simulink model "RefModel_FlightPerf"  (R2020b)
settings: Solver=ode1  StartTime=0.0  StopTime=10.0  FixedStep=SimParam.FightPerf.Ts_base  RelTol=1e-3
(part 2 of 2)

== stateflow chart RefModel_FlightPerf/FlightPerformanceModel/FlightPerf_StateFlow ==
  state FlightPerfPlatform [parallel]
    en:
    initMember();
    initOutputData();
    en,du:
    getTaskData();
    getFlightData();
    getWindData();
    getMavData();
    settings: executionOrder=1
    state LogData [parallel]
      en:
      settings: executionOrder=1
      state Work
        en,du:
        du_func_commonInfo();
        du_func_updateLog();
      (default) -> FlightPerfPlatform.LogData.Work
    state Core [parallel]
      settings: executionOrder=2
      state PowerConsumeByUavMode [parallel]
        settings: executionOrder=1
        state Rotor
          en:
        state Fix
          en:
        (default) -> FlightPerfPlatform.Core.PowerConsumeByUavMode.Rotor
        FlightPerfPlatform.Core.PowerConsumeByUavMode.Rotor -> Fix : [isUavInFix]
        Fix -> FlightPerfPlatform.Core.PowerConsumeByUavMode.Rotor : [isUavInRotor]
      state OverAllParam [parallel]
        settings: executionOrder=2
        state Rotor
          en:
          initFlightPerOut;
          du:
          on every(ceil(0.2/Ts),tick):
          predictDistToFly;
          on every(ceil(1/Ts),tick):
          predictTimeAndPowerToFly(1);
          predictRemainPowerWhenComplete;
          isPowerEnoughToCompleteTask;
        (default) -> FlightPerfPlatform.Core.OverAllParam.Rotor
      state EconomicAirspeed [parallel]
        settings: executionOrder=3
        state Work
          en,du:
          du_func;
        (default) -> FlightPerfPlatform.Core.EconomicAirspeed.Work
  data: flag function_output; period function_input; flag function_output; lla function_input; ll0 function_input; p function_output; blockName function_input; message function_input; operation function_input; varargin function_input; success function_output; message_in function_input; varargin function_input; debugInfo function_input; tabspace function_input; varargin function_input; modeName function_input; debugInfo function_input; varargin function_input; clock_sec input; isDebugInfoToShow input; Ts input; IN_TaskCmd input Bus: BUS_TASK_PATH_OutParam size=1; IN_FlightParam input Bus: BUS_TASK_COMMON_OutParam size=1; mission_item_def input Bus: mavlink_mission_item_def size=TASK_PARAM_V1000.maxPathPointNum; TaskParam data_store_memory; FlightPerfParam data_store_memory size=1; FlightPerfOut output Bus: BUS_FLIGHTPERF_OUT size=1; mavlink_msg_command_battery_data input Bus: mavlink_msg_command_battery_data size=1; mavlink_msg_mission_current input Bus: mavlink_msg_mission_current; IN_WindNED input; TimeSpend local; logDataBuffer output Bus: BUS_FLIGHTPERF_SingleLog size=32; logDataOut output Bus: BUS_FLIGHTPERF_SingleLog size=1; mTask_taskMode local; mTask_currentPointNum local =2; mTask_validPathNum local; mTask_uavMode local; mTask_heightSwitchMode local; mFParam_LLA local; mFParam_WindSpeed local; mFParam_HomeLLA local; mFParam_altitude local; mWind_WindSpeed local; mWind_WindHeading local; mMav_batteryLife local =0
  function initOutputData:
    | function initOutputData
    | % 输出结构体进行赋值，避免报"调用前没有赋值"的错误，每个结构体赋值1个成员即可
    | logDataOut(1).time_sec = 0;
    | logDataBuffer(1).time_sec = 0;
  function initMember:
    | function initMember()
    | % 初始化成员变量
    | mTask_currentPointNum = 0;
    | mTask_validPathNum = 0;
  function getTaskData:
    | function getTaskData()
    | %% 输入结构体
    | %% 直接量
    | mTask_taskMode = IN_TaskCmd.flightTaskMode;
    | mTask_currentPointNum = IN_TaskCmd.currentPointNum;
    | mTask_validPathNum = IN_TaskCmd.validPathNum;
    | mTask_uavMode = IN_TaskCmd.uavMode;
    | mTask_heightSwitchMode = IN_TaskCmd.heightSwitchMode;
    | %% 间接量
  function getMavData:
    | function getMavData()
    | %% 输入结构体
    | %% 直接量
    | mMav_batteryLife = getLowestBatteryLife(); %double(mavlink_msg_mission_current(1).remaining);
    | %% 间接量
    | 
    | %% 子函数 ------------------------------------------------------------
    | function minLife = getLowestBatteryLife()
    | persistent du
    | if isempty(du)
    |     du = 0;
    | end
    | out = 0;
    | du = du + Ts;
    | nIter = TaskParam.maxNumBattery;
    | nValid = TaskParam.nBattery;
    | flagAllZero = true;
    | minLife = 100;
    | for i = 1:nIter
    |     if i <= nValid
    |         thisLife = double(mavlink_msg_mission_current(i).remaining);
    |         if thisLife > 1e-6 % 非零
    |             flagAllZero = false;
    |             minLife = min(minLife,thisLife);
    |         end
    |     end
    | end
    | % if flagAllZero && du > 1
    | %     du = 0;
    | %     runLog(ENUM_RTInfo_Task.BatteryInfo_AllZero,[0,0,0,0,0]);
    | % end
  function getFlightData:
    | function getFlightData()
    | %% 输入结构体
    | %% 直接量
    | mFParam_LLA = IN_FlightParam.curLLA;
    | mFParam_WindSpeed = IN_FlightParam.curWindSpeedFromHead;
    | mFParam_HomeLLA = IN_FlightParam.curHomeLLA;
    | mFParam_altitude = IN_FlightParam.altitude;
    | %% 间接量
  function getWindData:
    | function getWindData()
    | %% 输入结构体
    | %% 直接量
    | mWind_WindSpeed = IN_WindNED.windSpeed_ms;
    | mWind_WindHeading = IN_WindNED.windHeading_rad;
    | %% 间接量
  function du_func_commonInfo:
    | function du_func_commonInfo
  function du_func_updateLog:
    | function du_func_updateLog
    | updateLogDataBuffer(ENUM_FlightPerfLogBlockName.FPLOG_None,ENUM_RTInfo_FlightPerf(0),'read')
  function predictRemainPowerWhenComplete:
    | function predictRemainPowerWhenComplete()
    | FlightPerfOut.remainPowerWhenFinish_per = mMav_batteryLife - FlightPerfOut.batteryLifeToCompleteTask;
  function predictDistToFly:
    | function predictDistToFly
    | persistent hasTakeOff remainDistToGo_movsmooth hasBeginGoHome
    | if isempty(hasTakeOff)
    |     hasTakeOff = false;
    |     hasBeginGoHome = false;
    |     remainDistToGo_movsmooth = 0;
    | end
    | if mTask_validPathNum == 0
    |     FlightPerfOut.remainDistToGo_m = 0;
    |     return;
    | end
    | validNum = 0;
    | maxNum = length(mission_item_def);
    | % 
    | nanFlag = TaskParam.nanFlag;
    | if isDataRefresh(mission_item_def,maxNum,nanFlag) % 检测航点是否更新
    |     refreshFlag = true;
    | else
    |     refreshFlag = false;
    | end
    | % 当前目标航点
    | if mTask_currentPointNum ~= 0 % 进入航线模式前
    |     idxCur = mTask_currentPointNum;
    | else
    |     idxCur = 2;
    | end
    | curPathPoint = double([mission_item_def(idxCur).x,mission_item_def(idxCur).y, mission_item_def(idxCur).z]);
    | % 最后一个航点
    | if mTask_validPathNum ~= 0
    |     idxLast = mTask_validPathNum;
    | else
    |     idxLast = 3;
    | end
    | lastValidPathPoint = double([mission_item_def(idxLast).x,mission_item_def(idxLast).y, mission_item_def(idxLast).z]);
    | % home点
    | idxHome = 1;
    | homePoint = double([mission_item_def(idxHome).x,mission_item_def(idxHome).y, mission_item_def(idxHome).z]);
    | % 当前位置
    | curLLA = mFParam_LLA;
    | %
    | % FlightPerfOut.remainDistToGo_m = 0;
    | if mTask_taskMode == ENUM_FlightTaskMode.TakeOffMode
    |     hasTakeOff = true;
    | end
    | if mTask_taskMode == ENUM_FlightTaskMode.GoHomeMode
    |     hasBeginGoHome = true;
    | end
    | %
    | switch mTask_taskMode
    |     case ENUM_FlightTaskMode.GroundStandByMode
    |         if hasTakeOff
    |             FlightPerfOut.remainDistToGo_m = 0;
    |         else
    |             idxStart = 1;
    |             restAllPath = calDistFromCurToHome(idxCur,maxNum,mTask_validPathNum,mission_item_def,FlightPerfParam,refreshFlag);
    |             tempPos = lla2ned(curLLA, curPathPoint(1:2));
    |             distToCurPathPoint = norm(tempPos(1:2));
    |             tempPos = lla2ned(lastValidPathPoint, homePoint(1:2));
    |             distFromEndPointToHome = norm(tempPos(1:2));
    |             FlightPerfOut.remainDistToGo_m = restAllPath + distToCurPathPoint + distFromEndPointToHome + 200;
    |         end
    |     case {  ENUM_FlightTaskMode.TakeOffMode,...
    |             ENUM_FlightTaskMode.HoverUpMode,...
    |             ENUM_FlightTaskMode.Rotor2Fix_Mode}
    |         modeflag = 'beforePathMode';
    |         idxStart = 1;
    |         restAllPath = calDistFromCurToHome(idxCur,maxNum,mTask_validPathNum,mission_item_def,FlightPerfParam,refreshFlag);
    |         tempPos = lla2ned(curLLA, curPathPoint(1:2));
    |         distToCurPathPoint = norm(tempPos(1:2));
    |         tempPos = lla2ned(lastValidPathPoint, homePoint(1:2));
    |         distFromEndPointToHome = norm(tempPos(1:2));
    |         FlightPerfOut.remainDistToGo_m = restAllPath + distToCurPathPoint + distFromEndPointToHome + 200;
    |     case {ENUM_FlightTaskMode.PathFollowMode,...
    |             ENUM_FlightTaskMode.AirStandByMode}
    |         modeflag = 'duringPathMode';
    |         idxStart = 2;
    |         restAllPath = calDistFromCurToHome(idxCur,maxNum,mTask_validPathNum,mission_item_def,FlightPerfParam,refreshFlag);
    |         tempPos = lla2ned(curLLA, curPathPoint(1:2));
    |         distToCurPathPoint = norm(tempPos(1:2));
    |         tempPos = lla2ned(lastValidPathPoint, homePoint(1:2));
    |         distFromEndPointToHome = norm(tempPos(1:2));
    |         FlightPerfOut.remainDistToGo_m = restAllPath + distToCurPathPoint + distFromEndPointToHome;
    |         if hasBeginGoHome && ...
    |                 mTask_taskMode == ENUM_FlightTaskMode.AirStandByMode
    |             FlightPerfOut.remainDistToGo_m = distToCurPathPoint;
    |         end
    |     case ENUM_FlightTaskMode.GoHomeMode
    |         modeflag = 'GoHomeMode';
    |         tempPos = lla2ned(curLLA, homePoint(1:2));
    |         distFromCurLLAToHome = norm(tempPos(1:2));
    |         FlightPerfOut.remainDistToGo_m = distFromCurLLAToHome;
    |     otherwise
    |         modeflag = 'afterHomeMode';
    | end
    | FlightPerfOut.remainDistToGo_m = movsmooth(FlightPerfOut.remainDistToGo_m);
    | end
    | %% 子函数
    | function flag = isDataRefresh(pathdata,maxNum,nanFlag)
    | persistent preSum
    | if isempty(preSum)
    |     preSum = 0;
    | end
    | flag = false;
    | sum = 0;
    | for i = 2:maxNum % 从第2个数据点开始，不考虑home点
    |     if pathdata(i).x ~= nanFlag
    |         sum = sum + double(i*pathdata(i).x + 1.1*i*pathdata(i).y);
    |     end
    | end
    | if preSum ~= sum
    |     flag = true;
    | end
    | preSum = sum;
    | end
    | 
    | function [remainDistToGo_m] = calDistFromCurToHome(curNum,maxNum,validNum,mission_item_def,FlightPerfParam,refreshFlag)
    | % 从当前位置算起，完成剩余航点后返回到home点的总距离
    |     persistent isPathValid isCalComplete pathDistSet
    |     if isempty(isPathValid)
    |         isPathValid = false;
    |         isCalComplete = false;
    |         pathDistSet = zeros(1,maxNum);
    |     end
    |     if validNum >= 2 && (~isCalComplete || refreshFlag) 
    |         isPathValid = true;
    |         for idx = curNum:maxNum-1
    |             tempPrePathPoint = double([mission_item_def(idx).x,mission_item_def(idx).y, mission_item_def(idx).z]);
    |             tempCurPathPoint = double([mission_item_def(idx+1).x,mission_item_def(idx+1).y, mission_item_def(idx+1).z]);
    |             tempPos = lla2ned(tempPrePathPoint, tempCurPathPoint(1:2));
    |             tempDist = norm(tempPos(1:2));
    |             if idx <= validNum-1
    |                 pathDistSet(idx) = tempDist;
    |             else
    |                 break;
    |             end
    |         end
    |         isCalComplete = true;
    |     end
    |     modeSel = 'pre_cal'; % rt_cal pre_cal  实时计算or预计算
    |     switch modeSel
    |         case 'rt_cal'
    |             if curNum ~= 0 % 进入航线模式前
    |                 idxCur = curNum;
    |             else
    |                 idxCur = 2;
    |             end
    |             curPathPoint = double([mission_item_def(idxCur).x,mission_item_def(idxCur).y, mission_item_def(idxCur).z]);
    |             remainDistToGo_m = 0;
    |             remainPathPoint = 0;
    |             for idx = curNum:maxNum-1
    |                 tempPrePathPoint = double([mission_item_def(idx).x,mission_item_def(idx).y, mission_item_def(idx).z]);
    |                 tempCurPathPoint = double([mission_item_def(idx+1).x,mission_item_def(idx+1).y, mission_item_def(idx+1).z]);
    |                 tempPos = lla2ned(tempPrePathPoint, tempCurPathPoint(1:2));
    |                 tempDist = norm(tempPos(1:2));
    |                 if idx <= validNum-1 && isPathPointValid(curPathPoint)
    |                     remainDistToGo_m = remainDistToGo_m + tempDist + FlightPerfParam.addedDistByEachTurnCorrect;
    |                 else
    |                     break;
    |                 end
    |             end
    |         otherwise
    |             nPoint = validNum - curNum;
    |             remainDistToGo_m = sum(pathDistSet(curNum:end)) + nPoint*FlightPerfParam.addedDistByEachTurnCorrect;
    |     end
    | end
    | %
    | function out = movsmooth(val)
    | persistent valsmooth
    | if isempty(valsmooth)
    |     valsmooth = 0;
    | end
    | if val ~= 0
    |     %     if norm(valsmooth-val)<2000
    |     kscale = 11/12;
    |     valsmooth = kscale*valsmooth + (1-kscale)*val;
    |     out = valsmooth;
    |     %     else
    |     %         out = val;
    |     %     end
    | else
    |     out = 0;
    | end
    | end
    | %
    | function flag = isPathPointValid(LLA)
    | flag = true;
    | for i_LLA = 1:2
    |     if abs(LLA(i_LLA)) > 360
    |         flag = false;
    |     end
    | end
    | end
  function flag = isUavInRotor:
    | function flag = isUavInRotor
    | flag = false;
    | if mTask_uavMode == ENUM_UAVMode.Rotor
    |     flag = true;
    | end
  function isPowerEnoughToCompleteTask:
    | function isPowerEnoughToCompleteTask
    | if FlightPerfOut.remainPowerWhenFinish_per <= FlightPerfParam.reservedPowerRate_normal %TaskParam.low_battery_alarm_set
    |     FlightPerfOut.isAbleToCompleteTask = false;
    | else 
    |     FlightPerfOut.isAbleToCompleteTask = true;
    | end
  function predictTimeAndPowerToFly(period):
    | function predictTimeAndPowerToFly(period)
    | persistent preTimeSpend preBatterySpend hasEnterLandMode hasEnterHoverDown hasBeenInPath hasVerticalMoveBeforePath hasVerticalMoveBeforeHome
    | if isempty(preTimeSpend)
    |     preTimeSpend = 0;
    |     preBatterySpend = 0;
    |     hasEnterHoverDown = false;
    |     hasEnterLandMode = false;
    |     hasBeenInPath = false;
    |     hasVerticalMoveBeforePath = false;
    |     hasVerticalMoveBeforeHome = false;
    | end
    | if FlightPerfOut.remainDistToGo_m == 0
    |     FlightPerfOut.remainTimeToSpend_sec = 0;
    |     return;
    | end
    | % 海拔、风等因素对续航的修正系数
    | k_Alt = calHeightScaleForPowerConsum();
    | kTakeOff_AltCorrect = 1.15*k_Alt;
    | kPath_AltCorrect = 1.15*k_Alt;
    | kLand_AltCorrect = 1.15*k_Alt;
    | kLand_WindCorrect = 1+abs(mWind_WindSpeed)/15; % 当风速15m/s时, 系数为 2
    | %
    | timeSpend = 0; % 完成任务所需时间
    | 
    | switchHeight = mTask_heightSwitchMode; % 固定翼切换高度
    | curHeight = mFParam_LLA(3);
    | homeHeight = double(mission_item_def(1).z); % home高度，注意，等高航线中home点高度存在高于航线高度的情况
    | pathHeight = double(mission_item_def(2).z); % 航线高度 ！V1000仅有等高航线，若后续增加变高航线，该处可能需调整
    | errHeight_Home_Path = abs(homeHeight-pathHeight);
    | errHeight_Cur_Path = abs(curHeight-pathHeight);
    | errHeight_Cur_Home = abs(curHeight-homeHeight);
    | % 模式耗时
    | timeSpend_TakeOff = 15 + switchHeight/(TaskParam.maxClimbSpeed_normal_TakeOffandLand+eps);
    | timeSpend_HoverAfterTakeOff = 10;
    | timeSpend_Rotor2Fix = 10;
    | timeSpend_HoverUp = abs(homeHeight-switchHeight)/(TaskParam.maxClimbSpeed_fixMode+eps);
    | timeSpend_VerticalMoveBeforePath = errHeight_Home_Path/(TaskParam.maxClimbSpeed_fixMode+eps);
    | timeSpend_Path = FlightPerfOut.remainDistToGo_m/(TaskParam.cruiseSpeed_cruise+eps)+FlightPerfOut.remainPathPoint*15;
    | timeSpend_VerticalMoveBeforeGoHome = errHeight_Home_Path/(TaskParam.maxClimbSpeed_fixMode+eps);
    | timeSpend_HoverDown = timeSpend_HoverUp + 25;
    | timeSpend_Fix2Rotor = 10;
    | timeSpend_GoHome_Rotor_full = 100/TaskParam.cruiseSpeed_rotorMode;
    | timeSpend_GoHome_Rotor_part = FlightPerfOut.remainDistToGo_m/TaskParam.cruiseSpeed_rotorMode;
    | timeSpend_Land = kLand_WindCorrect*kLand_AltCorrect*timeSpend_TakeOff;
    | timeSpend_LandFromHomeHeight_ByRotor = kLand_WindCorrect*kLand_AltCorrect*curHeight/(TaskParam.maxClimbSpeed_normal_TakeOffandLand+eps);
    | 
    | batteryLifeSpend_TakeOff = kTakeOff_AltCorrect*timeSpend_TakeOff*FlightPerfParam.powerRate_RotorUpNoWind;
    | batteryLifeSpend_HoverAfterTakeOff = timeSpend_HoverAfterTakeOff*FlightPerfParam.powerRate_RotorHoverNoWind;
    | batteryLifeSpend_Rotor2Fix = timeSpend_Rotor2Fix*FlightPerfParam.powerRate_RotorHoverNoWind;
    | batteryLifeSpend_HoverUp = timeSpend_HoverUp*FlightPerfParam.powerRate_FixHoverUp;
    | batteryLifeSpend_VerticalMoveBeforePath = timeSpend_VerticalMoveBeforePath*FlightPerfParam.powerRate_FixHoverDown;
    | batteryLifeSpend_Path = kPath_AltCorrect*timeSpend_Path*FlightPerfParam.powerRate_FixCruise;
    | batteryLifeSpend_VerticalMoveBeforeGoHome = timeSpend_VerticalMoveBeforeGoHome*FlightPerfParam.powerRate_FixHoverUp;
    | batteryLifeSpend_HoverDown = timeSpend_HoverDown*FlightPerfParam.powerRate_FixHoverDown;
    | batteryLifeSpend_Fix2Rotor = timeSpend_Fix2Rotor*FlightPerfParam.powerRate_RotorUpNoWind;
    | batteryLifeSpend_GoHome_Rotor_full = timeSpend_GoHome_Rotor_full*FlightPerfParam.powerRate_RotorMoveNoWind;
    | batteryLifeSpend_GoHome_Rotor_part = timeSpend_GoHome_Rotor_part*FlightPerfParam.powerRate_RotorMoveNoWind;
    | batteryLifeSpend_Land = timeSpend_Land*FlightPerfParam.powerRate_RotorDownNoWind;
    | batteryLifeSpend_LandFromHomeHeight_ByRotor = timeSpend_LandFromHomeHeight_ByRotor*FlightPerfParam.powerRate_RotorDownNoWind;
    | 
    | if mTask_taskMode == ENUM_FlightTaskMode.LandMode
    |     hasEnterLandMode = true;
    | end
    | if mTask_taskMode == ENUM_FlightTaskMode.HoverDownMode
    |     hasEnterHoverDown = true;
    | end
    | if mTask_taskMode == ENUM_FlightTaskMode.VerticalMove
    |     hasVerticalMoveBeforePath = true;
    | end
    | if mTask_currentPointNum > 2
    |     hasBeenInPath = true;
    | end
    | if mTask_taskMode == ENUM_FlightTaskMode.VerticalMove && hasBeenInPath
    |     hasVerticalMoveBeforeHome = true;
    | end
    | switch mTask_taskMode
    |     case ENUM_FlightTaskMode.GroundStandByMode
    |         if hasEnterLandMode
    |             timeSpend = 0;
    |             batterySpend = 0;
    |         else
    |             timeSpend = ...
    |                 timeSpend_TakeOff + ...
    |                 timeSpend_HoverAfterTakeOff + ...
    |                 timeSpend_Rotor2Fix + ...
    |                 timeSpend_HoverUp + ...
    |                 timeSpend_VerticalMoveBeforePath + ...
    |                 timeSpend_Path + ...
    |                 timeSpend_VerticalMoveBeforeGoHome + ...
    |                 timeSpend_HoverDown + ...
    |                 timeSpend_Fix2Rotor + ...
    |                 timeSpend_GoHome_Rotor_full + ...
    |                 timeSpend_Land;
    |             batterySpend = ...
    |                 batteryLifeSpend_TakeOff + ...
    |                 batteryLifeSpend_HoverAfterTakeOff + ...
    |                 batteryLifeSpend_Rotor2Fix + ...
    |                 batteryLifeSpend_HoverUp + ...
    |                 batteryLifeSpend_VerticalMoveBeforePath + ...
    |                 batteryLifeSpend_Path + ...
    |                 batteryLifeSpend_VerticalMoveBeforeGoHome + ...
    |                 batteryLifeSpend_HoverDown + ...
    |                 batteryLifeSpend_Fix2Rotor + ...
    |                 batteryLifeSpend_GoHome_Rotor_full + ...
    |                 batteryLifeSpend_Land;
    |         end
    |     case ENUM_FlightTaskMode.TakeOffMode
    |         timeSpend = ...
    |             timeSpend_Rotor2Fix + ...
    |             timeSpend_HoverUp + ...
    |             timeSpend_VerticalMoveBeforePath + ...
    |             timeSpend_Path + ...
    |             timeSpend_VerticalMoveBeforeGoHome + ...
    |             timeSpend_HoverDown + ...
    |             timeSpend_Fix2Rotor + ...
    |             timeSpend_GoHome_Rotor_full + ...
    |             timeSpend_Land;
    |         batterySpend = ...
    |             batteryLifeSpend_Rotor2Fix + ...
    |             batteryLifeSpend_HoverUp + ...
    |             batteryLifeSpend_VerticalMoveBeforePath + ...
    |             batteryLifeSpend_Path + ...
    |             batteryLifeSpend_VerticalMoveBeforeGoHome + ...
    |             batteryLifeSpend_HoverDown + ...
    |             batteryLifeSpend_Fix2Rotor + ...
    |             batteryLifeSpend_GoHome_Rotor_full + ...
    |             batteryLifeSpend_Land;
    |         timeByThisTask = 10 + max(0,switchHeight-curHeight)/(TaskParam.maxClimbSpeed_normal_TakeOffandLand+eps);
    |         timeSpend = timeSpend + timeByThisTask;
    |         batterySpendByThisTask = kTakeOff_AltCorrect*timeByThisTask*FlightPerfParam.powerRate_RotorUpNoWind;
    |         batterySpend = batterySpend + batterySpendByThisTask;
    |     case ENUM_FlightTaskMode.HoverUpMode
    |         timeSpend = ...
    |             timeSpend_VerticalMoveBeforePath + ...
    |             timeSpend_Path + ...
    |             timeSpend_VerticalMoveBeforeGoHome + ...
    |             timeSpend_HoverDown + ...
    |             timeSpend_Fix2Rotor + ...
    |             timeSpend_GoHome_Rotor_full + ...
    |             timeSpend_Land;
    |         batterySpend = ...
    |             batteryLifeSpend_VerticalMoveBeforePath + ...
    |             batteryLifeSpend_Path + ...
    |             batteryLifeSpend_VerticalMoveBeforeGoHome + ...
    |             batteryLifeSpend_HoverDown + ...
    |             batteryLifeSpend_Fix2Rotor + ...
    |             batteryLifeSpend_GoHome_Rotor_full + ...
    |             batteryLifeSpend_Land;
    |         timeByThisTask = 10 + max(0,homeHeight-curHeight)/(TaskParam.maxClimbSpeed_fixMode+eps);
    |         timeSpend = timeSpend + timeByThisTask;
    |         batterySpendByThisTask = timeByThisTask*FlightPerfParam.powerRate_FixHoverUp;
    |         batterySpend = batterySpend + batterySpendByThisTask;
    |     case ENUM_FlightTaskMode.VerticalMove
    |         if hasVerticalMoveBeforePath && ~hasVerticalMoveBeforeHome
    |             % 从home高度降至path高度
    |             timeSpend = ...
    |                 timeSpend_Path + ...
    |                 timeSpend_VerticalMoveBeforeGoHome + ...
    |                 timeSpend_HoverDown + ...
    |                 timeSpend_Fix2Rotor + ...
    |                 timeSpend_GoHome_Rotor_full + ...
    |                 timeSpend_Land;
    |             timeSpend_VerticalMoveBeforePath_RT = errHeight_Cur_Path/(TaskParam.maxClimbSpeed_fixMode+eps);
    |             timeSpend = timeSpend + timeSpend_VerticalMoveBeforePath_RT;
    |             batterySpend = ...
    |                 batteryLifeSpend_Path + ...
    |                 batteryLifeSpend_VerticalMoveBeforeGoHome + ...
    |                 batteryLifeSpend_HoverDown + ...
    |                 batteryLifeSpend_Fix2Rotor + ...
    |                 batteryLifeSpend_GoHome_Rotor_full + ...
    |                 batteryLifeSpend_Land;
    |             batterySpend = batterySpend + timeSpend_VerticalMoveBeforePath_RT*FlightPerfParam.powerRate_FixHoverDown;
    |         else % if hasVerticalMoveBeforePath
    |             % 从path高度上升至home高度
    |             timeSpend = ...
    |                 timeSpend_Path + ...
    |                 timeSpend_HoverDown + ...
    |                 timeSpend_Fix2Rotor + ...
    |                 timeSpend_GoHome_Rotor_full + ...
    |                 timeSpend_Land;
    |             timeSpend_VerticalMoveBeforeGoHome_RT = errHeight_Cur_Home/(TaskParam.maxClimbSpeed_fixMode+eps);
    |             timeSpend = timeSpend + timeSpend_VerticalMoveBeforeGoHome_RT;
    |             batterySpend = ...
    |                 batteryLifeSpend_Path + ...
    |                 batteryLifeSpend_HoverDown + ...
    |                 batteryLifeSpend_Fix2Rotor + ...
    |                 batteryLifeSpend_GoHome_Rotor_full + ...
    |                 batteryLifeSpend_Land;
    |             batterySpend = batterySpend + timeSpend_VerticalMoveBeforeGoHome_RT*FlightPerfParam.powerRate_FixHoverUp;
    |         end
    |     case ENUM_FlightTaskMode.PathFollowMode
    |         timeSpend = ...
    |             timeSpend_Path + ...
    |             timeSpend_HoverDown + ...
    |             timeSpend_Fix2Rotor + ...
    |             timeSpend_GoHome_Rotor_full + ...
    |             timeSpend_Land;
    |         batterySpend = ...
    |             batteryLifeSpend_Path + ...
    |             batteryLifeSpend_HoverDown + ...
    |             batteryLifeSpend_Fix2Rotor + ...
    |             batteryLifeSpend_GoHome_Rotor_full + ...
    |             batteryLifeSpend_Land;
    |         if ~hasVerticalMoveBeforePath
    |             timeSpend = timeSpend + timeSpend_VerticalMoveBeforePath + timeSpend_VerticalMoveBeforeGoHome;
    |             batterySpend = batterySpend + ...
    |                 batteryLifeSpend_VerticalMoveBeforePath + ...
    |                 batteryLifeSpend_VerticalMoveBeforeGoHome;
    |         elseif hasVerticalMoveBeforePath && ~hasVerticalMoveBeforeHome
    |             timeSpend_VerticalMoveBeforePath_RT = errHeight_Cur_Path/(TaskParam.maxClimbSpeed_fixMode+eps);
    |             timeSpend = timeSpend + timeSpend_VerticalMoveBeforePath_RT + timeSpend_VerticalMoveBeforeGoHome;
    |             batterySpend = batterySpend + ...
    |                 timeSpend_VerticalMoveBeforePath_RT*FlightPerfParam.powerRate_FixHoverDown + ...
    |                 batteryLifeSpend_VerticalMoveBeforeGoHome;
    |         elseif hasVerticalMoveBeforeHome
    |             timeSpend_VerticalMoveBeforeGoHome_RT = errHeight_Cur_Home/(TaskParam.maxClimbSpeed_fixMode+eps);
    |             timeSpend = timeSpend + timeSpend_VerticalMoveBeforeGoHome_RT;
    |             batterySpend = batterySpend + ...
    |                 timeSpend_VerticalMoveBeforeGoHome_RT*FlightPerfParam.powerRate_FixHoverDown;
    |         end
    |     case ENUM_FlightTaskMode.GoHomeMode
    |         if ~hasEnterHoverDown
    |             timeSpend = ...
    |                 timeSpend_Path + ...
    |                 timeSpend_HoverDown + ...
    |                 timeSpend_Fix2Rotor + ...
    |                 timeSpend_GoHome_Rotor_full + ...
    |                 timeSpend_Land;
    |             batterySpend = ...
    |                 batteryLifeSpend_Path + ...
    |                 batteryLifeSpend_HoverDown + ...
    |                 batteryLifeSpend_Fix2Rotor + ...
    |                 batteryLifeSpend_GoHome_Rotor_full + ...
    |                 batteryLifeSpend_Land;
    |         else
    |             timeSpend = ...
    |                 timeSpend_GoHome_Rotor_part + ...
    |                 timeSpend_Land;
    |             batterySpend = ...
    |                 batteryLifeSpend_GoHome_Rotor_part + ...
    |                 batteryLifeSpend_Land;
    |         end
    |     case ENUM_FlightTaskMode.HoverDownMode
    |         if abs(curHeight-switchHeight) > 10
    |             % 盘旋下降（不考虑滑翔方式的节能影响，让按照正常耗电计算）
    |             timeSpend = ...
    |                 timeSpend_Fix2Rotor + ...
    |                 timeSpend_GoHome_Rotor_full + ...
    |                 timeSpend_Land;
    |             batterySpend = ...
    |                 batteryLifeSpend_Fix2Rotor + ...
    |                 batteryLifeSpend_GoHome_Rotor_full + ...
    |                 batteryLifeSpend_Land;
    |             timeByThisTask = abs(curHeight-switchHeight)/(TaskParam.maxClimbSpeed_fixMode+eps)+20;
    |             timeSpend = timeSpend + timeByThisTask;
    |             batterySpendByThisTask = timeByThisTask*FlightPerfParam.powerRate_FixHoverDown;
    |             batterySpend = batterySpend + batterySpendByThisTask;
    |         else
    |             % 盘旋一圈
    |             timeSpend = preTimeSpend - period;
    |             batterySpend = preBatterySpend - period*FlightPerfParam.powerRate_FixHoverLevel;
    |         end
    |     case ENUM_FlightTaskMode.LandMode
    |         if curHeight-10 > 0
    |             timeSpend = (curHeight-10)/(TaskParam.maxClimbSpeed_normal_TakeOffandLand+eps) + 10/TaskParam.maxClimbSpeed_nearGround_TakeOffandLand;
    |         else
    |             timeSpend = curHeight/TaskParam.maxClimbSpeed_nearGround_TakeOffandLand;
    |         end
    |         batterySpend = timeSpend*FlightPerfParam.powerRate_RotorDownNoWind;
    |     case ENUM_FlightTaskMode.Fix2Rotor_Mode
    |         timeSpend = preTimeSpend - period;
    |         batterySpend = preBatterySpend - period*FlightPerfParam.powerRate_RotorHoverNoWind;
    |     case ENUM_FlightTaskMode.Rotor2Fix_Mode
    |         timeSpend = preTimeSpend - period;
    |         batterySpend = preBatterySpend - period*FlightPerfParam.powerRate_RotorHoverNoWind;
    |     case {ENUM_FlightTaskMode.HoverAdjustMode,...
    |             ENUM_FlightTaskMode.AirStandByMode}
    |         timeSpend = preTimeSpend;
    |         batterySpend = preBatterySpend;
    |     otherwise
    |         timeSpend = preTimeSpend;
    |         batterySpend = preBatterySpend;
    | end
    | %% 电量低返航触发标志
    | % 计算风因素对飞行地速的影响
    | homeLLA = mFParam_HomeLLA;
    | curLLA = mFParam_LLA;
    | homeNED = lla2ned(homeLLA,curLLA);
    | curLLA = [0 0 0];
    | headingGoHome_rad = atan2(homeNED(2),homeNED(1));
    | headingErr = angdiff(mWind_WindHeading,headingGoHome_rad);
    | windSpeedWhenGoHomeAtThisLL = mWind_WindSpeed*cos(headingErr); % 正值表示逆风, 负值表示顺风
    | windSpeedWhenGoHomeAtThisLL = min(windSpeedWhenGoHomeAtThisLL,14); % 限制小于14
    | windSpeedWhenGoHomeAtThisLL = max(windSpeedWhenGoHomeAtThisLL,-5); % 限制大于-5
    | 
    | velScale_FixGoHome = 1;
    | speedmode = 'fixAirspeed';
    | switch speedmode
    |     case 'fixAirspeed'
    |         velScale_FixGoHome = TaskParam.cruiseSpeed_cruise / abs(TaskParam.cruiseSpeed_cruise-windSpeedWhenGoHomeAtThisLL);
    | %         velScale_FixGoHome1 = TaskParam.cruiseSpeed_cruise / abs(TaskParam.cruiseSpeed_cruise-windSpeedWhenGoHomeAtThisLL1);
    | %         fprintf('(%.2f) velScale_FixGoHome: %.2f\t\tvelScale_FixGoHome1: %.2f\n',clock_sec,velScale_FixGoHome,velScale_FixGoHome1);
    |     case 'variableAirspeed'
    |         velScale_FixGoHome = 1 + windSpeedWhenGoHomeAtThisLL/TaskParam.cruiseSpeed_cruise;
    | end
    | velScale_RotorGoHome = velScale_FixGoHome;
    | % 注意"盘旋下降、降落、固定翼转旋翼"不进行判断，因为盘旋下降已经处于降落流程且盘旋下降模式耗电量极低
    | % if mTask_taskMode == ENUM_FlightTaskMode.PathFollowMode || ...
    | %         mTask_taskMode == ENUM_FlightTaskMode.GoHomeMode || ...
    | %         mTask_taskMode == ENUM_FlightTaskMode.AirStandByMode || ...
    | %         mTask_taskMode == ENUM_FlightTaskMode.HoverAdjustMode
    | if mTask_taskMode ~= ENUM_FlightTaskMode.GroundStandByMode && ...
    |         mTask_taskMode ~= ENUM_FlightTaskMode.HoverDownMode && ...
    |         mTask_taskMode ~= ENUM_FlightTaskMode.Rotor2Fix_Mode && ...
    |         mTask_taskMode ~= ENUM_FlightTaskMode.LandMode && ...
    |         mTask_taskMode ~= ENUM_FlightTaskMode.NoneFlightTaskMode
    |     % 计算当前点到Home点距离
    |     curLLA = mFParam_LLA;
    |     idxHome = 1;
    |     homeLLA = double([mission_item_def(idxHome).x,mission_item_def(idxHome).y, mission_item_def(idxHome).z]);
    |     tempPos = lla2ned(curLLA, homeLLA(1:2));
    |     distFromCurToHome = norm(tempPos(1:2));
    |     [FlightPerfOut.batterylifeNeededToHome,FlightPerfOut.batterylifeNeededToLand] = batteryLifeToHome(distFromCurToHome,mTask_uavMode,...
    |         batteryLifeSpend_HoverDown,batteryLifeSpend_Fix2Rotor,batteryLifeSpend_GoHome_Rotor_full,batteryLifeSpend_Land,batteryLifeSpend_LandFromHomeHeight_ByRotor,velScale_FixGoHome,velScale_RotorGoHome);
    |     extraLifeNeededByWind = 1/3*abs(mWind_WindSpeed);
    |     if (FlightPerfOut.batterylifeNeededToHome + extraLifeNeededByWind) >= mMav_batteryLife - FlightPerfParam.reservedPowerRate_normal
    |         FlightPerfOut.flagGoHomeNow = true;
    | %         if isDebugInfoToShow
    | %             fprintf('%.3f sec: [flagGoHomeNow] TaskMode(%d) ',clock_sec,mTask_taskMode,) 
    | %         end
    |     end
    |     if (FlightPerfOut.batterylifeNeededToLand + extraLifeNeededByWind) >= mMav_batteryLife - FlightPerfParam.reservedPowerRate_rotor && ...
    |             mTask_uavMode == ENUM_UAVMode.Rotor % (mTask_uavMode == ENUM_UAVMode.Rotor || mTask_uavMode == ENUM_UAVMode.Fix)
    |         % 目前仅在旋翼模式下判断该值，存在逻辑缺陷
    |         FlightPerfOut.flagLandNow = true;
    |     end
    | end
    | %%
    | FlightPerfOut.remainTimeToSpend_sec = double(timeSpend);
    | FlightPerfOut.batteryLifeToCompleteTask = double(batterySpend);
    | preTimeSpend = double(FlightPerfOut.remainTimeToSpend_sec);
    | preBatterySpend = FlightPerfOut.batteryLifeToCompleteTask;
    | end
    | %% 子函数
    | % 计算耗电系数的海拔修正
    | function out = calHeightScaleForPowerConsum()
    | persistent pK_height
    | if isempty(pK_height)
    |     pK_height = 1;
    | end
    | k_height = 1 + FlightPerfParam.powerRatio_Altitude*abs(mFParam_altitude/6e3);
    | % 0.9 < k_height < 1.5
    | k_height = min(k_height,2); % < 2
    | k_height = max(k_height,0.9); % > 0.9
    | tempK = 0.95;
    | pK_height = tempK*pK_height + (1-tempK)*k_height;
    | out = pK_height;
    | end
    | % 计算立即返航所需电量
    | function [batterySpendToHome,batterySpendToLand] = batteryLifeToHome(distFromCurToHome,uavMode,...
    |     batteryLifeSpend_HoverDown,batteryLifeSpend_Fix2Rotor,batteryLifeSpend_GoHome_Rotor_full,batteryLifeSpend_Land,batteryLifeSpend_LandFromHomeHeight_ByRotor,velScale_FixGoHome,velScale_RotorGoHome)
    | if uavMode == ENUM_UAVMode.Fix
    |     batteryLifeSpend_ToHome = velScale_FixGoHome*distFromCurToHome/(TaskParam.cruiseSpeed_cruise+eps)*FlightPerfParam.powerRate_FixCruise;
    |     batterySpendToLand = ...
    |         batteryLifeSpend_HoverDown + ...
    |         batteryLifeSpend_Fix2Rotor + ...
    |         batteryLifeSpend_GoHome_Rotor_full + ...
    |         batteryLifeSpend_Land;
    |     batterySpendToHome = ...
    |         batteryLifeSpend_ToHome + ...
    |         batterySpendToLand;
    | else
    |     batteryLifeSpend_ToHome = velScale_RotorGoHome*distFromCurToHome/(TaskParam.cruiseSpeed_rotorMode-0.5+eps)*FlightPerfParam.powerRate_RotorMoveNoWind;
    |     batterySpendToLand = batteryLifeSpend_LandFromHomeHeight_ByRotor;
    |     batterySpendToHome = ...
    |         batteryLifeSpend_ToHome + ...
    |         batterySpendToLand;
    | end
    | 
    | end
  function flag = isUavInFix:
    | function flag = isUavInFix
    | flag = false;
    | if mTask_uavMode == ENUM_UAVMode.Fix
    |     flag = true;
    | end
  function p = lla2ned(lla, ll0):
    | function p = lla2ned(lla, ll0)
    | % 纬经高转换为NED位置
    | % lla: 纬度[deg] 经度[deg] 高度[m] 
    | % ll0: 基准点， 纬度[deg] 经度[deg]
    | % p: NED位置
    | p = zeros(1,3);
    | psi0 = 0;
    | href = 0;
    | f = 0.003352810664747;
    | R = 6378.137e3;
    | % wrap latitude and longitude if needed
    | [~, lla(:,1), lla(:,2)] = wraplatitude( lla(:,1), lla(:,2), 'deg' );
    | [~, ll0(1), ll0(2)] = wraplatitude( ll0(1), ll0(2), 'deg' );
    | 
    | % check and fix angle wrapping in longitude
    | [~, lla(:,2)] = wraplongitude( lla(:,2), 'deg', '180' );
    | [~, ll0(2)] = wraplongitude( ll0(2), 'deg', '180' );
    | 
    | dLat = lla(:,1) - ll0(1);
    | dLon = lla(:,2) - ll0(2);
    | 
    | % wrap latitude and longitude if needed
    | [~, dLat, dLon] = wraplatitude( dLat', dLon', 'deg' );
    | 
    | % check and fix angle wrapping in longitude
    | [~, dLon] = wraplongitude( dLon, 'deg', '180' );
    | 
    | rll0 = ll0*pi/180;
    | rpsi0 = psi0*pi/180;
    | 
    | Rn = R/sqrt(1-(2*f-f*f)*sin(rll0(1))*sin(rll0(1)));
    | Rm = Rn*((1-(2*f-f*f))/(1-(2*f-f*f)*sin(rll0(1))*sin(rll0(1))));
    | 
    | dNorth = dLat./atan2(1,Rm)*pi/180;
    | dEast = dLon./atan2(1,Rn*cos(rll0(1)))*pi/180;
    | 
    | p(:,1) = cos(rpsi0)*dNorth + sin(rpsi0)*dEast;
    | p(:,2) = -sin(rpsi0)*dNorth + cos(rpsi0)*dEast;
    | p(:,3) = -lla(:,3) - href;
    | end
    | 
    | function [lat_wrapped, lat, lon] = wraplatitude( lat, lon, units)
    | % WRAPLATITUDE internal function to check and fix angle wrapping in
    | % latitude and longitude if needed.
    | 
    | %   Copyright 2007-2013 The MathWorks, Inc.
    | 
    | % Convert units if necessary
    | if strcmp(units,'deg')
    |     pideg = 180;
    | else
    |     pideg = pi;
    | end
    | 
    | % Set lat_wrapped flag to false
    | lat_wrapped = false;
    | 
    | % Re-set latitudes to values between pi and -pi
    | flat = abs(lat);
    | 
    | if any(flat>pideg)
    |     lat(flat>pideg) = mod(lat(flat>pideg)+pideg,2*pideg)-pideg;
    |     % Set lat_wrapped flag to true if necessary
    |     flat = abs(lat);
    |     lat_wrapped = true;
    | end
    | 
    | % Determine if any latitudes need to be wrapped
    | idx = flat>pideg/2;
    | 
    | if any(idx)
    |     
    |     % Adjustments for -pi to pi
    |     flat = abs(lat);
    |     latp2 = flat>pideg/2;
    |     lon(idx) = lon(idx) + pideg;
    |     lat(latp2) = sign(lat(latp2)).*(pideg/2-(flat(latp2)-pideg/2));
    |     
    |     % Set lat_wrapped flag to true if necessary
    |     lat_wrapped = true;
    |     
    | end
    | end
    | 
    | function [lon_wrapped, lon] = wraplongitude( lon, inputUnits, maxRange )
    | % WRAPLONGITUDE internal function to check and fix angle wrapping in
    | % longitude.
    | 
    | %   Copyright 2007-2010 The MathWorks, Inc.
    | 
    | % Convert units if necessary
    | if strcmp(inputUnits,'deg')
    |     lon = lon*pi/180;
    | end
    | 
    | lon_wrapped = false;
    | 
    | switch maxRange
    |     % Range goes between -pi and pi
    |     case {'180','pi'}
    |         idx = lon > pi | lon < -pi;
    |         if any(idx)
    |             lon(idx) = rem(lon(idx),2*pi)- (2*pi)*fix(rem(lon(idx),2*pi)/pi);
    |             lon_wrapped = true;
    |         end
    |     % Range goes between 0 and 2*pi
    |     case {'360','2*pi'}
    |         idx = lon > 2*pi | lon < 0;
    |         if any(idx)
    |             lon(idx) = mod(lon(idx),2*pi);
    |             lon_wrapped = true;
    |         end
    |     otherwise
    |         % do nothing
    | end
    | 
    | % Convert units if necessary
    | if strcmp(inputUnits,'deg')
    |     lon = lon*180/pi;
    | end
    | end
  function initFlightPerOut:
    | function initFlightPerOut
    | FlightPerfOut.isAbleToCompleteTask = true;
    | FlightPerfOut.remainDistToGo_m = 0;
    | FlightPerfOut.remainTimeToSpend_sec = 0;
    | FlightPerfOut.remainPowerWhenFinish_per = 0;
  function du_func:
    | function du_func
    | persistent smoothVal
    | if isempty(smoothVal)
    |     smoothVal = TaskParam.minAirspeed_fixAllowed;
    | end
    | % 空速指令应大于最小允许空速
    | temp = TaskParam.minAirspeed_fixAllowed;
    | % 地速指令应等于XX （地速 = 空速-风速>XX  空速>XX+风速）
    | % temp = max(temp,mFParam_WindSpeed+TaskParam.cruiseSpeed_cruise);
    | temp = max(temp,mFParam_WindSpeed+15);
    | k = 0.85;
    | smoothVal = k*smoothVal + (1-k)*temp;
    | FlightPerfOut.economicAirspeed = max(TaskParam.minAirspeed_fixAllowed,smoothVal);
  function updateLogDataBuffer(blockName,message,operation,varargin):
    | function updateLogDataBuffer(blockName,message,operation,varargin)
    | persistent pIdx pBufferIdx preTime
    | if isempty(pIdx)
    |     pIdx = 0;
    |     pBufferIdx = 0;
    |     preTime = clock_sec;
    | end
    | %%
    | if nargin == 4
    |     var_input = double(reshape(varargin{1},5,1));
    | else
    |     var_input = zeros(5,1);
    | end
    | bufferIdx = pBufferIdx;
    | idx = pIdx;
    | switch operation
    |     case 'write'
    |         thisTime = clock_sec;
    |         if preTime ~= thisTime
    |             idx = 0; % 同一时间刻度下, 不同信息的先后顺序
    |         end
    |         preTime = thisTime;
    |         if bufferIdx < length(logDataBuffer)
    |             bufferIdx = bufferIdx + 1;
    |             idx = idx + 1;
    |             temp = formatLogStruct(blockName,message,var_input);
    |             tempData.time_sec = clock_sec;
    |             tempData.idx = idx;
    |             tempData.blockName = blockName;
    |             tempData.message = message;
    |             tempData.var1 = temp.var1;
    |             logDataBuffer(bufferIdx) = tempData;            
    |         end
    |     case 'read'
    |         for i_out = 1:1 %AlgoParams.logDataOutSize
    |             %             logDataOut(i_out) = resetLogStruct; % 置零
    |             logDataOut(i_out).time_sec = 0;
    |             logDataOut(i_out).idx = 0;
    |             logDataOut(i_out).blockName = ENUM_FlightPerfLogBlockName(0);
    |             logDataOut(i_out).message = ENUM_RTInfo_FlightPerf(0);
    |             logDataOut(i_out).var1 = zeros(5,1);
    |             if bufferIdx > 0
    |                 % 读取当前数据
    |                 logDataOut(i_out) = logDataBuffer(bufferIdx);
    |                 %                 logDataBuffer(bufferIdx) = resetLogStruct;
    | %                 fprintf('read time \t idx \t block \t message \t var1\n%.3f \t %.0f \t %d \t %d \t %.3f\n',...
    | %                     logDataBuffer(bufferIdx).time_sec,...
    | %                     logDataBuffer(bufferIdx).idx,...
    | %                     int16(logDataBuffer(bufferIdx).blockName),...
    | %                     int16(logDataBuffer(bufferIdx).message),...
    | %                     logDataBuffer(bufferIdx).var1(1));
    |                 % 将当前位置数据置零
    |                 logDataBuffer(bufferIdx).time_sec = 0;
    |                 logDataBuffer(bufferIdx).idx = 0;
    |                 logDataBuffer(bufferIdx).blockName = ENUM_FlightPerfLogBlockName(0);
    |                 logDataBuffer(bufferIdx).message = ENUM_RTInfo_FlightPerf(0);
    |                 logDataBuffer(bufferIdx).var1 = zeros(5,1);
    |                 bufferIdx = bufferIdx - 1;
    |             end
    |         end
    | end
    | % fprintf("logbuffer  %d / %d\n", int16(bufferIdx), int16(length(logDataBuffer)));
    | pBufferIdx = bufferIdx;
    | pIdx = idx;
    | %% 子函数
    | function log = formatLogStruct(blockName,message,var_input)
    | log.message = message;
    | log.var1 = zeros(5,1);
    | % switch blockName
    | %     case ENUM_TaskLogBlockName.TASKLOG_FlightMode
    | %         log.var1(1) = ComFlightOut.curLLA(1);
    | %         log.var1(2) = ComFlightOut.curLLA(2);
    | %         log.var1(3) = ComFlightOut.curLLA(3);
    | %         log.var1(4) = norm(ComFlightOut.curAirSpeed);
    | %         log.var1(5) = PathModeOut.uavMode;
    | % end
    | % log.var1(5) = double(IN_Mav.mavlink_msg_mission_current(1).remaining)/100;
    | if sum(var_input) ~= 0
    |     log.var1 = var_input; % 输入的优先级高
    | end
  function success = runLog(message_in,varargin):
    | function success = runLog(message_in,varargin)
    | if nargin == 2
    |     var_input = varargin{1};
    | else
    |     var_input = zeros(5,1);
    | end
    | success = true;
    | switch message_in
    |     %% GoHome 模块
    |     case ENUM_RTInfo_Navi.RTIN_InitWait_1_Complete
    |         mThis_RTInfo = message_in; % 更新RT信息
    |         updateLogDataBuffer(ENUM_NaviLogBlockName.NAVILOG_Init,mThis_RTInfo,'write',var_input); % 更新log缓存
    |     case ENUM_RTInfo_Navi.RTIN_InitWait_2_Complete
    |         mThis_RTInfo = message_in; % 更新RT信息
    |         updateLogDataBuffer(ENUM_NaviLogBlockName.NAVILOG_Init,mThis_RTInfo,'write',var_input); % 更新log缓存
    |     case ENUM_RTInfo_Navi.RTIN_Init_Complete
    |         mThis_RTInfo = message_in; % 更新RT信息
    |         updateLogDataBuffer(ENUM_NaviLogBlockName.NAVILOG_Init,mThis_RTInfo,'write',var_input); % 更新log缓存
    |         %% coarseAlignment
    |     case ENUM_RTInfo_Navi.RTIN_Init_Enter
    |         mThis_RTInfo = message_in; % 更新RT信息
    |         updateLogDataBuffer(ENUM_NaviLogBlockName.NAVILOG_Init,mThis_RTInfo,'write',var_input); % 更新log缓存
    |         %% MARG22
    |     case ENUM_RTInfo_Navi.RTIN_Filter_Init
    |         mThis_RTInfo = message_in; % 更新RT信息
    |         updateLogDataBuffer(ENUM_NaviLogBlockName.NAVILOG_Marg22,mThis_RTInfo,'write',var_input); % 更新log缓存
    |     case ENUM_RTInfo_Navi.RTIN_Filter_Param1
    |         mThis_RTInfo = message_in; % 更新RT信息
    |         updateLogDataBuffer(ENUM_NaviLogBlockName.NAVILOG_Marg22,mThis_RTInfo,'write',var_input); % 更新log缓存
    |     case ENUM_RTInfo_Navi.RTIN_Filter_Fuse_Mag
    |         mThis_RTInfo = message_in; % 更新RT信息
    |         updateLogDataBuffer(ENUM_NaviLogBlockName.NAVILOG_Marg22,mThis_RTInfo,'write',var_input); % 更新log缓存
    |     case ENUM_RTInfo_Navi.RTIN_Filter_Fuse_Ublox
    |         mThis_RTInfo = message_in; % 更新RT信息
    |         updateLogDataBuffer(ENUM_NaviLogBlockName.NAVILOG_Marg22,mThis_RTInfo,'write',var_input); % 更新log缓存
    |     case ENUM_RTInfo_Navi.RTIN_Filter_Fuse_Um482
    |         mThis_RTInfo = message_in; % 更新RT信息
    |         updateLogDataBuffer(ENUM_NaviLogBlockName.NAVILOG_Marg22,mThis_RTInfo,'write',var_input); % 更新log缓存
    |     case ENUM_RTInfo_Navi.RTIN_Filter_GPSVelErrorLarge
    |         mThis_RTInfo = message_in; % 更新RT信息
    |         updateLogDataBuffer(ENUM_NaviLogBlockName.NAVILOG_Marg22,mThis_RTInfo,'write',var_input); % 更新log缓存
    |     case ENUM_RTInfo_Navi.RTIN_Filter_Fuse_Baro
    |         mThis_RTInfo = message_in; % 更新RT信息
    |         updateLogDataBuffer(ENUM_NaviLogBlockName.NAVILOG_Marg22,mThis_RTInfo,'write',var_input); % 更新log缓存
    |     case ENUM_RTInfo_Navi.RTIN_Filter_Fuse_Airspeed
    |         mThis_RTInfo = message_in; % 更新RT信息
    |         updateLogDataBuffer(ENUM_NaviLogBlockName.NAVILOG_Marg22,mThis_RTInfo,'write',var_input); % 更新log缓存
    |     otherwise
    |         success = false;
    |         fprintf('FlightPerf Log Error: No Message ID %d\n',int32(message_in));
    | end
  function printComInfo(debugInfo,tabspace,varargin):
    | function printComInfo(debugInfo,tabspace,varargin)
    | if nargin == 3
    |     value = double(varargin{1});
    |     noValue = false;
    | else
    |     value = 0;
    |     noValue = true;
    | end
    | if isDebugInfoToShow
    |     if ~noValue
    |         switch tabspace
    |             case 0
    |                 fprintf([' %.3f sec: ',debugInfo,'\n'],clock_sec,value);
    |             case 1
    |                 fprintf(['\t %.3f sec: ',debugInfo,'\n'],clock_sec,value);
    |             case 2
    |                 fprintf(['\t\t %.3f sec: ',debugInfo,'\n'],clock_sec,value);
    |             case 3
    |                 fprintf(['\t\t\t %.3f sec: ',debugInfo,'\n'],clock_sec,value);
    |             case 4
    |                 fprintf(['\t\t\t\t %.3f sec: ',debugInfo,'\n'],clock_sec,value);
    |         end
    |     else
    |         switch tabspace
    |             case 0
    |                 fprintf([' %.3f sec: ',debugInfo,'\n'],clock_sec);
    |             case 1
    |                 fprintf(['\t %.3f sec: ',debugInfo,'\n'],clock_sec);
    |             case 2
    |                 fprintf(['\t\t %.3f sec: ',debugInfo,'\n'],clock_sec);
    |             case 3
    |                 fprintf(['\t\t\t %.3f sec: ',debugInfo,'\n'],clock_sec);
    |             case 4
    |                 fprintf(['\t\t\t\t %.3f sec: ',debugInfo,'\n'],clock_sec);
    |         end        
    |     end
    | end
  function printDebugInfo(modeName,debugInfo,varargin):
    | function printDebugInfo(modeName,debugInfo,varargin)
    | if nargin == 3
    |     tabspace = varargin{1};
    | else
    |     tabspace = 2;
    | end
    | if isDebugInfoToShow
    |     switch tabspace
    |         case 0
    |             fprintf(' %.3f sec: [%s] %s\n',clock_sec,modeName,debugInfo);
    |         case 1
    |             fprintf('\t %.3f sec: [%s] %s\n',clock_sec,modeName,debugInfo);
    |         case 2
    |             fprintf('\t\t %.3f sec: [%s] %s\n',clock_sec,modeName,debugInfo);
    |         case 3
    |             fprintf('\t\t\t %.3f sec: [%s] %s\n',clock_sec,modeName,debugInfo);
    |         case 4
    |             fprintf('\t\t\t\t %.3f sec: [%s] %s\n',clock_sec,modeName,debugInfo);
    |     end
    | end
